simulink model "EngineCtrl_V2"  (R2018a)
settings: Solver=VariableStepAuto  StartTime=0.0  StopTime=10.0  FixedStep=sampletime  RelTol=1e-3  EnableMultiTasking=on
PreLoadFcn:
  | EngineCtrl_V1_1_BusInfo
libraries: simulink x2
settings Model: Creator=IAEC nishito  LastModifiedBy=nishito
settings DataIOCC: LimitDataPoints=on  SaveFormat=Array  SignalLoggingSaveFormat=ModelDataLogs  SaveOutput=off  SaveTime=off
settings OptimizationCC: DefaultParameterBehavior=Inlined  ExpressionDepthLimit=2147483647  LifeSpan=inf
settings DebuggingCC: SolverPrmCheckMsg=warning  FcnCallInpInsideContextMsg=warning  StateNameClashWarn=warning  SFUnexpectedBacktrackingDiag=warning  SFNoUnconditionalDefaultTransitionDiag=warning  SFExecutionAtInitializationDiag=none
settings HardwareCC: ProdBitPerPointer=32  ProdBitPerSizeT=32  ProdBitPerPtrDiffT=32  ProdLargestAtomicFloat=None  ProdIntDivRoundTo=Undefined  ProdEndianess=Unspecified  ProdWordSize=32  ProdHWDeviceType=32-bit Generic
settings ModelReferenceCC: UpdateModelReferenceTargets=IfOutOfDate  PropagateSignalLabelsOutOfModel=off
settings CodeAppCC: StateflowObjectComments=on
settings GRTTargetCC: TargetLangStandard=C89/C90 (ANSI)  GeneratePreprocessorConditionals=Disable all  CombineOutputUpdateFcns=off  GRTInterface=on
settings ConfigComp: CovMetricSettings=dw  CovHtmlReporting=on  CovSaveCumulativeToWorkspaceVar=on  CovSaveSingleToWorkspaceVar=on  CovExternalEMLEnable=off

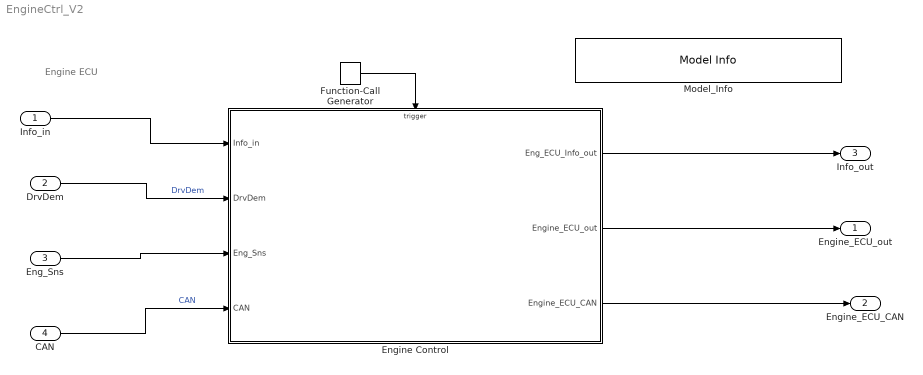
== system EngineCtrl_V2 ==
  note: Engine ECU
  Info_in : Inport  OutDataTypeStr=Bus: Engine_ECU_Info_in_Bus
      settings: AttributesFormatString=%<OutDataTypeStr>
  DrvDem : Inport  Port=2  OutDataTypeStr=Bus: Driver_demand_Bus
      settings: AttributesFormatString=%<OutDataTypeStr>
  Eng_Sns : Inport  Port=3  OutDataTypeStr=Bus: Engine_sensor_Bus
      settings: AttributesFormatString=%<OutDataTypeStr>
  CAN : Inport  Port=4  OutDataTypeStr=Bus: CAN_Bus
      settings: AttributesFormatString=<%<OutDataTypeStr>>
  Engine Control : Subsystem
  Function-Call Generator : simulink/Ports & Subsystems/Function-Call Generator  sample_time=0.01  numberOfIterations=1
      settings: AttributesFormatString=<sample_time=%<sample_time>>
  Model_Info : simulink/Model-Wide Utilities/Model Info  Frame=on  DisplayStringWithTags=|  HorizontalTextAlignment=Left  LeftAlignmentValue=0.02
      | Version  %<ModelVersion>
      | LastModifided by %<LastModifiedBy>  Date %<LastModificationDate>
      | Description  %<Description>
  Engine_ECU_out : Outport  OutDataTypeStr=Bus: Engine_ECU_out_Bus  BusOutputAsStruct=on
      settings: AttributesFormatString=<%<OutDataTypeStr>>
  Engine_ECU_CAN : Outport  Port=2  OutDataTypeStr=Bus: Engine_ECU_CAN_Bus  BusOutputAsStruct=on
      settings: AttributesFormatString=<%<OutDataTypeStr>>
  Info_out : Outport  Port=3  OutDataTypeStr=Bus: Engine_ECU_Info_out_Bus  BusOutputAsStruct=on
      settings: AttributesFormatString=<%<OutDataTypeStr>>
  wires:
  CAN/1 -> Engine Control/4(CAN)  "CAN"
  DrvDem/1 -> Engine Control/2(DrvDem)  "DrvDem"
  Eng_Sns/1 -> Engine Control/3(Eng_Sns)
  Function-Call Generator/1 -> Engine Control/Trigger
  Engine Control/3(Engine_ECU_CAN) -> Engine_ECU_CAN/1
  Engine Control/2(Engine_ECU_out) -> Engine_ECU_out/1
  Engine Control/1(Eng_ECU_Info_out) -> Info_out/1
  Info_in/1 -> Engine Control/1(Info_in)

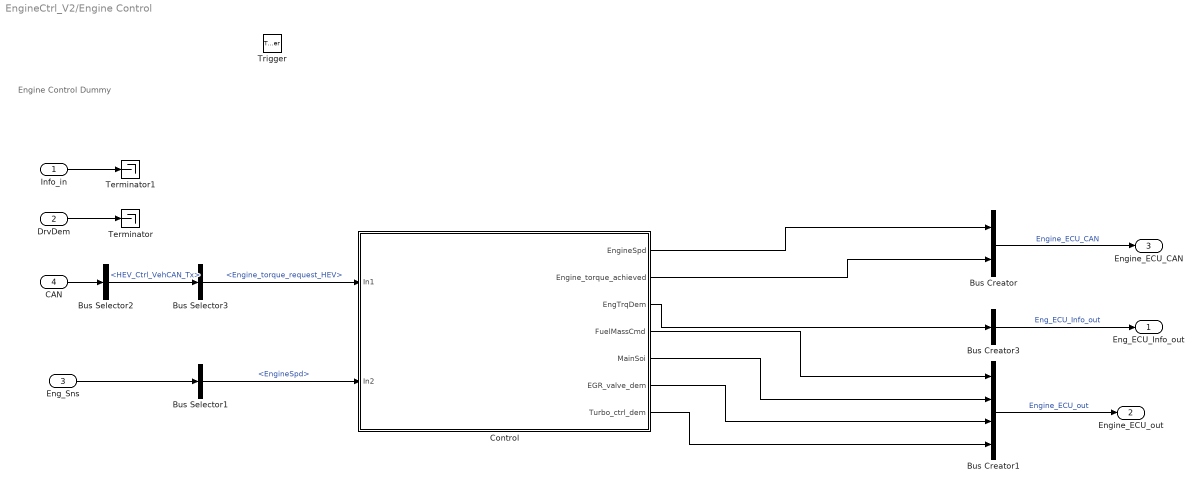
== system EngineCtrl_V2/Engine Control ==
  note: Engine Control Dummy
  Info_in : Inport
  DrvDem : Inport  Port=2
  Eng_Sns : Inport  Port=3
  CAN : Inport  Port=4
  Trigger : TriggerPort  TriggerType=function-call  VariantControl=Variant  PortDimensions=1
  Bus Creator : BusCreator  Inputs=2  OutDataTypeStr=Bus: Engine_ECU_CAN_Bus
      settings: AttributesFormatString=%<OutDataTypeStr>
  Bus Creator1 : BusCreator  Inputs=4  OutDataTypeStr=Bus: Engine_ECU_out_Bus
      settings: AttributesFormatString=%<OutDataTypeStr>
  Bus Creator3 : BusCreator  Inputs=1  OutDataTypeStr=Bus: Engine_ECU_Info_out_Bus
      settings: AttributesFormatString=%<OutDataTypeStr>
  Bus Selector1 : BusSelector  OutputSignals=EngineSpd
  Bus Selector2 : BusSelector  OutputSignals=VehCAN.HEV_Ctrl_VehCAN_Tx
  Bus Selector3 : BusSelector  OutputSignals=Engine_torque_request_HEV
  Control : Subsystem
  Terminator : Terminator
  Terminator1 : Terminator
  Eng_ECU_Info_out : Outport
  Engine_ECU_out : Outport  Port=2
  Engine_ECU_CAN : Outport  Port=3
  wires:
  DrvDem/1 -> Terminator/1
  CAN/1 -> Bus Selector2/1
  Eng_Sns/1 -> Bus Selector1/1
  Bus Creator/1 -> Engine_ECU_CAN/1  "Engine_ECU_CAN"
  Bus Creator1/1 -> Engine_ECU_out/1  "Engine_ECU_out"
  Bus Selector2/1 -> Bus Selector3/1  "<HEV_Ctrl_VehCAN_Tx>"
  Bus Selector3/1 -> Control/1(In1)  "<Engine_torque_request_HEV>"
  Bus Selector1/1 -> Control/2(In2)  "<EngineSpd>"
  Control/1(EngineSpd) -> Bus Creator/1
  Control/2(Engine_torque_achieved) -> Bus Creator/2
  Control/3(EngTrqDem) -> Bus Creator3/1
  Control/4(FuelMassCmd) -> Bus Creator1/1
  Control/7(Turbo_ctrl_dem) -> Bus Creator1/4
  Control/6(EGR_valve_dem) -> Bus Creator1/3
  Control/5(MainSoi) -> Bus Creator1/2
  Info_in/1 -> Terminator1/1
  Bus Creator3/1 -> Eng_ECU_Info_out/1  "Eng_ECU_Info_out"

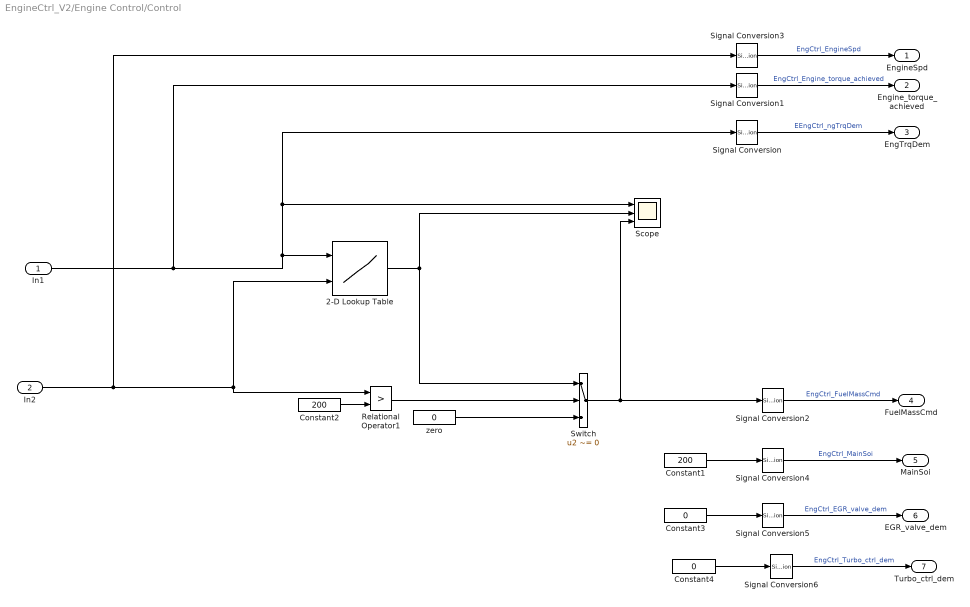
== system EngineCtrl_V2/Engine Control/Control ==
  In1 : Inport
  In2 : Inport  Port=2
  2-D Lookup Table : Lookup_n-D  BreakpointsForDimension1=[0 400]  BreakpointsForDimension2=[0 200 600 1000]  Table=[0 10 0 0; 70 70 70 70]  InternalRulePriority=Speed  RndMeth=Simplest  InputSameDT=on
  Constant1 : Constant  Value=200
  Constant2 : Constant  Value=200
  Constant3 : Constant  Value=0
  Constant4 : Constant  Value=0
  Relational Operator1 : RelationalOperator  Operator=>  OutDataTypeStr=boolean  RndMeth=Nearest
  Scope : Scope  NumInputPorts=3
  Signal Conversion{,1..6} (7 alike) : SignalConversion  OverrideOpt=off
  Switch : Switch  Criteria=u2 ~= 0  Threshold=0.5  SaturateOnIntegerOverflow=on
      settings: AttributesFormatString=<%<Criteria>>
  zero : Constant  Value=0
  EngineSpd : Outport
  Engine_torque_achieved : Outport  Port=2
  EngTrqDem : Outport  Port=3
  FuelMassCmd : Outport  Port=4
  MainSoi : Outport  Port=5
  EGR_valve_dem : Outport  Port=6
  Turbo_ctrl_dem : Outport  Port=7
  wires:
  Relational Operator1/1 -> Switch/2
  Signal Conversion3/1 -> EngineSpd/1  "EngCtrl_EngineSpd"
  zero/1 -> Switch/3
  Signal Conversion2/1 -> FuelMassCmd/1  "EngCtrl_FuelMassCmd"
  In1/1 -> Signal Conversion1/1, 2-D Lookup Table/1, Signal Conversion/1, Scope/1
  In2/1 -> Signal Conversion3/1, 2-D Lookup Table/2, Relational Operator1/1
  Signal Conversion1/1 -> Engine_torque_achieved/1  "EngCtrl_Engine_torque_achieved"
  Switch/1 -> Scope/3, Signal Conversion2/1
  Constant2/1 -> Relational Operator1/2
  Signal Conversion/1 -> EngTrqDem/1  "EEngCtrl_ngTrqDem"
  2-D Lookup Table/1 -> Switch/1, Scope/2
  Signal Conversion4/1 -> MainSoi/1  "EngCtrl_MainSoi"
  Constant1/1 -> Signal Conversion4/1
  Signal Conversion5/1 -> EGR_valve_dem/1  "EngCtrl_EGR_valve_dem"
  Constant3/1 -> Signal Conversion5/1
  Signal Conversion6/1 -> Turbo_ctrl_dem/1  "EngCtrl_Turbo_ctrl_dem"
  Constant4/1 -> Signal Conversion6/1
